simulink model "xfl_em2"  (R2019b)
settings: Solver=FixedStepAuto  StartTime=0  StopTime=50  FixedStep=1e-3  RelTol=1e-3  EnableMultiTasking=on
undefined symbols (not defined in the file or in its folder): qc
libraries: simulink x1
settings Model: Creator=acsl  LastModifiedBy=shawinmihail
settings DataIOCC: LimitDataPoints=on  ReturnWorkspaceOutputs=off
settings OptimizationCC: LifeSpan=inf
settings DebuggingCC: AllowSymbolicDim=off  SFUnexpectedBacktrackingDiag=warning  SFNoUnconditionalDefaultTransitionDiag=warning  SFExecutionAtInitializationDiag=none  ArithmeticOperatorsInVariantConditions=warning
settings ModelReferenceCC: PropagateSignalLabelsOutOfModel=off
settings SFSimCC: SimUseLocalCustomCode=off  CustomCodeUndefinedFunction=UseInterfaceOnly
settings RTWCC: RTWUseLocalCustomCode=off
settings CodeAppCC: StateflowObjectComments=on
settings GRTTargetCC: TargetLangStandard=C89/C90 (ANSI)
settings ConfigComp: CovMetricSettings=dw  CovHtmlReporting=on  CovSaveCumulativeToWorkspaceVar=on  CovSaveSingleToWorkspaceVar=on  CovExternalEMLEnable=off
settings SimscapeCC: SimscapeNormalizeSystem=off
settings ConfigurationSet: Description=SimMechanics 2G

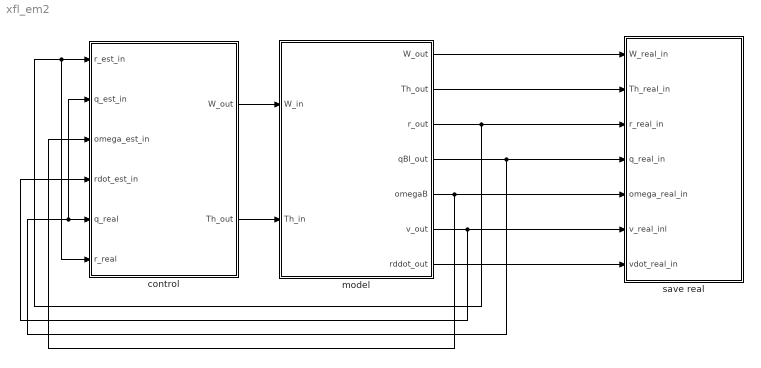
== system xfl_em2 ==
  control : Subsystem  InitFcn=init
  model : Subsystem
  save real : Subsystem
  wires:
  model/2(Th_out) -> save real/2(Th_real_in)
  model/7(rddot_out) -> save real/7(vdot_real_in)
  model/5(omegaB) -> control/3(omega_est_in), save real/5(omega_real_in)
  control/1(W_out) -> model/1(W_in)
  control/2(Th_out) -> model/2(Th_in)
  model/3(r_out) -> control/6(r_real), control/1(r_est_in), save real/3(r_real_in)
  model/4(qBI_out) -> control/5(q_real), control/2(q_est_in), save real/4(q_real_in)
  model/6(v_out) -> control/4(rdot_est_in), save real/6(v_real_inl)
  model/1(W_out) -> save real/1(W_real_in)

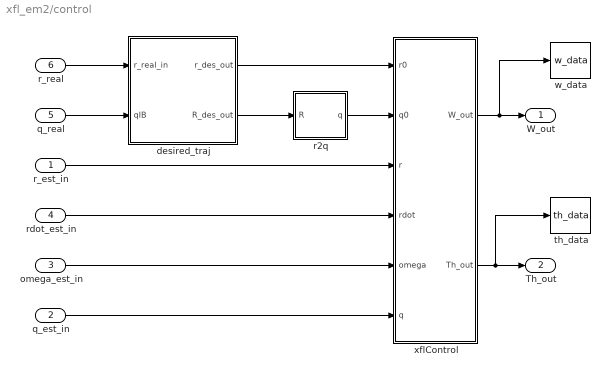
== system xfl_em2/control ==
  r_est_in : Inport
  q_est_in : Inport  Port=2
  omega_est_in : Inport  Port=3
  rdot_est_in : Inport  Port=4
  q_real : Inport  Port=5
  r_real : Inport  Port=6
  desired_traj : Subsystem
  r2q : MATLAB Function  TreatAsAtomicUnit=on
  th_data : ToWorkspace  VariableName=th_data  SaveFormat=Timeseries  SampleTime=-1
  w_data : ToWorkspace  VariableName=w_data  SaveFormat=Timeseries  SampleTime=-1
  xflControl : Subsystem
  W_out : Outport
  Th_out : Outport  Port=2
  wires:
  omega_est_in/1 -> xflControl/5(omega)
  q_est_in/1 -> xflControl/6(q)
  rdot_est_in/1 -> xflControl/4(rdot)
  r_est_in/1 -> xflControl/3(r)
  desired_traj/1(r_des_out) -> xflControl/1(r0)
  desired_traj/2(R_des_out) -> r2q/1(R)
  xflControl/1(W_out) -> w_data/1, W_out/1
  xflControl/2(Th_out) -> th_data/1, Th_out/1
  r2q/1(q) -> xflControl/2(q0)
  r_real/1 -> desired_traj/1(r_real_in)
  q_real/1 -> desired_traj/2(qIB)

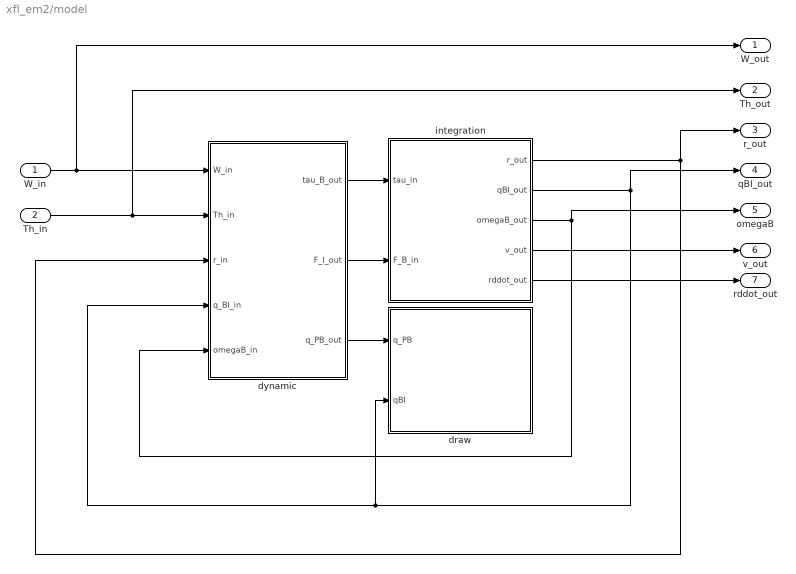
== system xfl_em2/model ==
  W_in : Inport
  Th_in : Inport  Port=2
  draw : Subsystem
  dynamic : Subsystem  StopFcn=close all
  integration : Subsystem
  W_out : Outport
  Th_out : Outport  Port=2
  r_out : Outport  Port=3
  qBI_out : Outport  Port=4
  omegaB : Outport  Port=5
  v_out : Outport  Port=6
  rddot_out : Outport  Port=7
  wires:
  integration/1(r_out) -> dynamic/3(r_in), r_out/1
  dynamic/2(F_I_out) -> integration/2(F_B_in)
  integration/2(qBI_out) -> dynamic/4(q_BI_in), draw/2(qBI), qBI_out/1
  W_in/1 -> W_out/1, dynamic/1(W_in)
  dynamic/1(tau_B_out) -> integration/1(tau_in)
  integration/3(omegaB_out) -> dynamic/5(omegaB_in), omegaB/1
  Th_in/1 -> dynamic/2(Th_in), Th_out/1
  dynamic/3(q_PB_out) -> draw/1(q_PB)
  integration/4(v_out) -> v_out/1
  integration/5(rddot_out) -> rddot_out/1

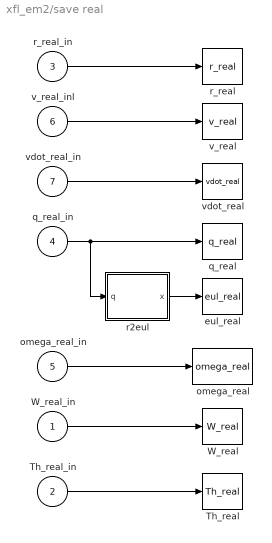
== system xfl_em2/save real ==
  W_real_in : Inport
  Th_real_in : Inport  Port=2
  r_real_in : Inport  Port=3
  q_real_in : Inport  Port=4
  omega_real_in : Inport  Port=5
  v_real_inl : Inport  Port=6
  vdot_real_in : Inport  Port=7
  Th_real : ToWorkspace  VariableName=Th_real  SaveFormat=Timeseries  SampleTime=-1
  W_real : ToWorkspace  VariableName=W_real  SaveFormat=Timeseries  SampleTime=-1
  eul_real : ToWorkspace  VariableName=eul_real  SaveFormat=Timeseries  SampleTime=-1
  omega_real : ToWorkspace  VariableName=omega_real  SaveFormat=Timeseries  SampleTime=-1
  q_real : ToWorkspace  VariableName=q_real  SaveFormat=Timeseries  SampleTime=-1
  r2eul : MATLAB Function  TreatAsAtomicUnit=on
  r_real : ToWorkspace  VariableName=r_real  SaveFormat=Timeseries  SampleTime=-1
  v_real : ToWorkspace  VariableName=v_real  SaveFormat=Timeseries  SampleTime=-1
  vdot_real : ToWorkspace  VariableName=vdot_real  SaveFormat=Timeseries  SampleTime=-1
  wires:
  q_real_in/1 -> q_real/1, r2eul/1(q)
  r_real_in/1 -> r_real/1
  v_real_inl/1 -> v_real/1
  vdot_real_in/1 -> vdot_real/1
  r2eul/1(x) -> eul_real/1
  omega_real_in/1 -> omega_real/1
  Th_real_in/1 -> Th_real/1
  W_real_in/1 -> W_real/1

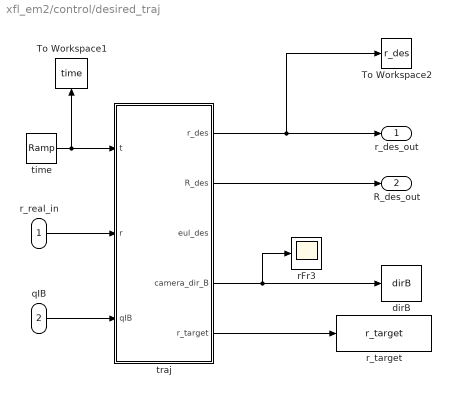
== system xfl_em2/control/desired_traj ==
  r_real_in : Inport
  qIB : Inport  Port=2
  To Workspace1 : ToWorkspace  VariableName=time  SaveFormat=Timeseries  SampleTime=-1
  To Workspace2 : ToWorkspace  VariableName=r_des  SaveFormat=Timeseries  SampleTime=-1
  dirB : ToWorkspace  VariableName=dirB  SaveFormat=Timeseries  SampleTime=-1
  rFr3 : Scope
  r_target : ToWorkspace  VariableName=r_target  SaveFormat=Timeseries  SampleTime=-1
  time : simulink/Sources/Ramp  slope=1  start=0  InitialOutput=0
  traj : MATLAB Function  TreatAsAtomicUnit=on
  r_des_out : Outport
  R_des_out : Outport  Port=2
  wires:
  traj/2(R_des) -> R_des_out/1
  time/1 -> traj/1(t), To Workspace1/1
  r_real_in/1 -> traj/2(r)
  traj/1(r_des) -> To Workspace2/1, r_des_out/1
  qIB/1 -> traj/3(qIB)
  traj/4(camera_dir_B) -> dirB/1, rFr3/1
  traj/5(r_target) -> r_target/1

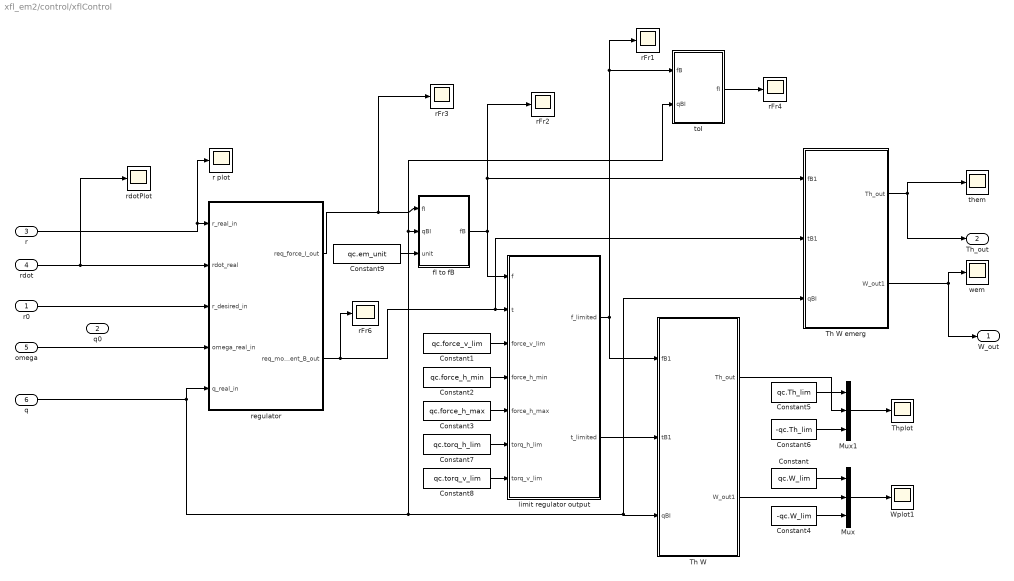
== system xfl_em2/control/xflControl ==
  r0 : Inport
  q0 : Inport  Port=2
  r : Inport  Port=3
  rdot : Inport  Port=4
  omega : Inport  Port=5
  q : Inport  Port=6
  Constant : Constant  Value=qc.W_lim
  Constant1 : Constant  Value=qc.force_v_lim
  Constant2 : Constant  Value=qc.force_h_min
  Constant3 : Constant  Value=qc.force_h_max
  Constant4 : Constant  Value=-qc.W_lim
  Constant5 : Constant  Value=qc.Th_lim
  Constant6 : Constant  Value=-qc.Th_lim
  Constant7 : Constant  Value=qc.torq_h_lim
  Constant8 : Constant  Value=qc.torq_v_lim
  Constant9 : Constant  Value=qc.em_unit
  Mux : Mux  Inputs=3
  Mux1 : Mux  Inputs=3
  Th W : Subsystem
  Th W emerg : Subsystem
  Thplot : Scope
  Wplot1 : Scope
  fI to fB : MATLAB Function  TreatAsAtomicUnit=on
  limit regulator output : MATLAB Function  TreatAsAtomicUnit=on
  r plot : Scope
  rFr{1..4,6} (5 alike) : Scope
  rdotPlot : Scope
  regulator : Subsystem
  them : Scope
  toI : MATLAB Function  TreatAsAtomicUnit=on
  wem : Scope
  W_out : Outport
  Th_out : Outport  Port=2
  wires:
  rdot/1 -> regulator/2(rdot_real), rdotPlot/1
  r0/1 -> regulator/3(r_desired_in)
  r/1 -> r plot/1, regulator/1(r_real_in)
  omega/1 -> regulator/4(omega_real_in)
  Th W/1(Th_out) -> Mux1/2
  Th W/2(W_out1) -> Mux/2
  regulator/1(req_force_I_out) -> rFr3/1, fI to fB/1(fI)
  regulator/2(req_moment_B_out) -> Th W emerg/2(tB1), limit regulator output/2(t), rFr6/1
  q/1 -> regulator/5(q_real_in), Th W emerg/3("qBI "), Th W/3("qBI "), toI/2(qBI), fI to fB/2(qBI)
  Constant/1 -> Mux/1
  Constant4/1 -> Mux/3
  Mux1/1 -> Thplot/1
  Constant5/1 -> Mux1/1
  Constant6/1 -> Mux1/3
  limit regulator output/2(t_limited) -> Th W/2(tB1)
  limit regulator output/1(f_limited) -> toI/1(fB), rFr1/1, Th W/1(fB1)
  Constant1/1 -> limit regulator output/3(force_v_lim)
  Constant2/1 -> limit regulator output/4(force_h_min)
  Constant3/1 -> limit regulator output/5(force_h_max)
  Constant7/1 -> limit regulator output/6(torq_h_lim)
  Constant8/1 -> limit regulator output/7(torq_v_lim)
  fI to fB/1(fB) -> limit regulator output/1(f), rFr2/1, Th W emerg/1(fB1)
  toI/1(fI) -> rFr4/1
  Mux/1 -> Wplot1/1
  Th W emerg/1(Th_out) -> Th_out/1, them/1
  Th W emerg/2(W_out1) -> W_out/1, wem/1
  Constant9/1 -> fI to fB/3(unit)

== system xfl_em2/model/draw ==
  q_PB : Inport
  qBI : Inport  Port=2
  Constant : Constant  Value=qc.rays
  Constant1 : Constant  Value=qc.l
  Constant2 : Constant  Value=qc.draw_mode
  Rate Transition : RateTransition
  Rate Transition1 : RateTransition
  draw : MATLAB Function  TreatAsAtomicUnit=on  SystemSampleTime=qc.draw_tick
  wires:
  Constant1/1 -> draw/4(l)
  q_PB/1 -> Rate Transition1/1
  Rate Transition1/1 -> draw/2(q_PB)
  Constant/1 -> draw/3(rays)
  Rate Transition/1 -> draw/1(q_BI)
  qBI/1 -> Rate Transition/1
  Constant2/1 -> draw/5(draw_mode)

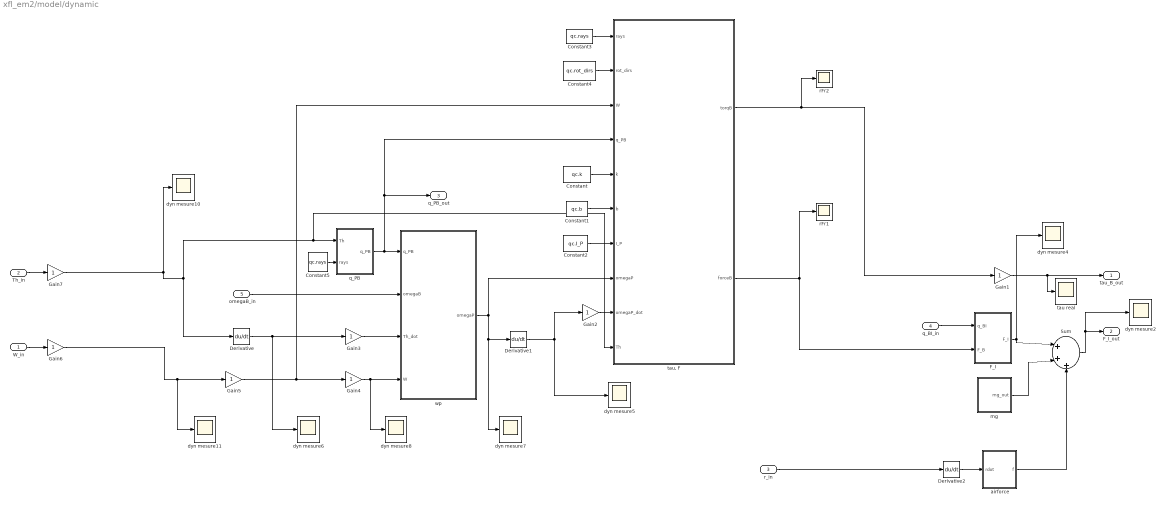
== system xfl_em2/model/dynamic ==
  W_in : Inport
  Th_in : Inport  Port=2
  r_in : Inport  Port=3
  q_BI_in : Inport  Port=4
  omegaB_in : Inport  Port=5
  Constant : Constant  Value=qc.k
  Constant1 : Constant  Value=qc.b
  Constant2 : Constant  Value=qc.I_P
  Constant3 : Constant  Value=qc.rays
  Constant4 : Constant  Value=qc.rot_dirs
  Constant5 : Constant  Value=qc.rays
  Derivative : Derivative
  Derivative1 : Derivative
  Derivative2 : Derivative
  F_I : MATLAB Function  TreatAsAtomicUnit=on
  Gain{1..7} (7 alike) : Gain
  Sum : Sum  Inputs=|+++
  airforce : Subsystem
  dyn mesure{2,4..8,10..11} (8 alike) : Scope
  mg : Subsystem
  q_PB : MATLAB Function  TreatAsAtomicUnit=on
  rFr1 : Scope
  rFr2 : Scope
  tau real : Scope
  "tau, F" : MATLAB Function  TreatAsAtomicUnit=on
  wp : MATLAB Function  TreatAsAtomicUnit=on
  tau_B_out : Outport
  F_I_out : Outport  Port=2
  q_PB_out : Outport  Port=3
  wires:
  q_PB/1(q_PB) -> "tau, F"/4(q_PB), q_PB_out/1, wp/1(q_PB)
  omegaB_in/1 -> wp/2(omegaB)
  Derivative/1 -> dyn mesure6/1, Gain3/1
  wp/1(omegaP) -> dyn mesure7/1, Derivative1/1, "tau, F"/8(omegaP)
  Constant/1 -> "tau, F"/5(k)
  Constant1/1 -> "tau, F"/6(b)
  Constant2/1 -> "tau, F"/7(I_P)
  Constant3/1 -> "tau, F"/1(rays)
  Constant4/1 -> "tau, F"/2(rot_dirs)
  Constant5/1 -> q_PB/2(rays)
  q_BI_in/1 -> F_I/1(q_BI)
  F_I/1(F_I) -> Sum/1, dyn mesure4/1
  mg/1(mg_out) -> Sum/2
  Sum/1 -> dyn mesure2/1, F_I_out/1
  r_in/1 -> Derivative2/1
  airforce/1(f) -> Sum/3
  Derivative2/1 -> airforce/1(rdot)
  Gain2/1 -> "tau, F"/9(omegaP_dot)
  Gain3/1 -> wp/3(Th_dot)
  Gain4/1 -> dyn mesure8/1, wp/4(W)
  Derivative1/1 -> dyn mesure5/1, Gain2/1
  Gain1/1 -> tau_B_out/1, tau real/1
  Gain5/1 -> "tau, F"/3(W), Gain4/1
  Gain6/1 -> dyn mesure11/1, Gain5/1
  Gain7/1 -> "tau, F"/10(Th), q_PB/1(Th), Derivative/1, dyn mesure10/1
  W_in/1 -> Gain6/1
  Th_in/1 -> Gain7/1
  "tau, F"/1(torqB) -> rFr2/1, Gain1/1
  "tau, F"/2(forceB) -> rFr1/1, F_I/2(F_B)

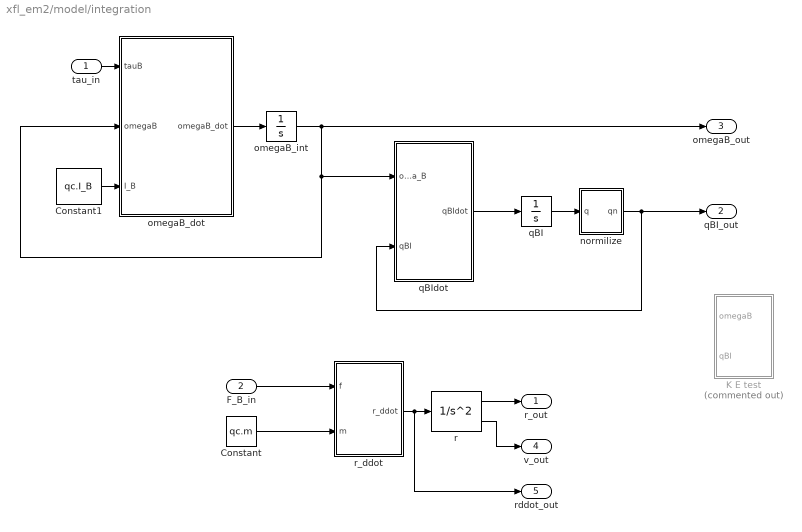
== system xfl_em2/model/integration ==
  tau_in : Inport
  F_B_in : Inport  Port=2
  Constant : Constant  Value=qc.m
  Constant1 : Constant  Value=qc.I_B
  K E test : Subsystem  Commented=on
  normilize : MATLAB Function  TreatAsAtomicUnit=on
  omegaB_dot : MATLAB Function  TreatAsAtomicUnit=on
  omegaB_int : Integrator  InitialCondition=qc.omegaB0
  qBI : Integrator  InitialCondition=qc.qBI0
  qBIdot : MATLAB Function  TreatAsAtomicUnit=on
  r : SecondOrderIntegrator  ICX=qc.r0  ICDXDT=qc.v0
  r_ddot : MATLAB Function  TreatAsAtomicUnit=on
  r_out : Outport
  qBI_out : Outport  Port=2
  omegaB_out : Outport  Port=3
  v_out : Outport  Port=4
  rddot_out : Outport  Port=5
  wires:
  r/1 -> r_out/1
  r_ddot/1(r_ddot) -> rddot_out/1, r/1
  Constant/1 -> r_ddot/2(m)
  omegaB_int/1 -> omegaB_out/1, qBIdot/1(omega_B), omegaB_dot/2(omegaB)
  Constant1/1 -> omegaB_dot/3(I_B)
  tau_in/1 -> omegaB_dot/1(tauB)
  qBIdot/1(qBIdot) -> qBI/1
  qBI/1 -> normilize/1(q)
  normilize/1(qn) -> qBI_out/1, qBIdot/2(qBI)
  F_B_in/1 -> r_ddot/1(f)
  omegaB_dot/1(omegaB_dot) -> omegaB_int/1
  r/2 -> v_out/1

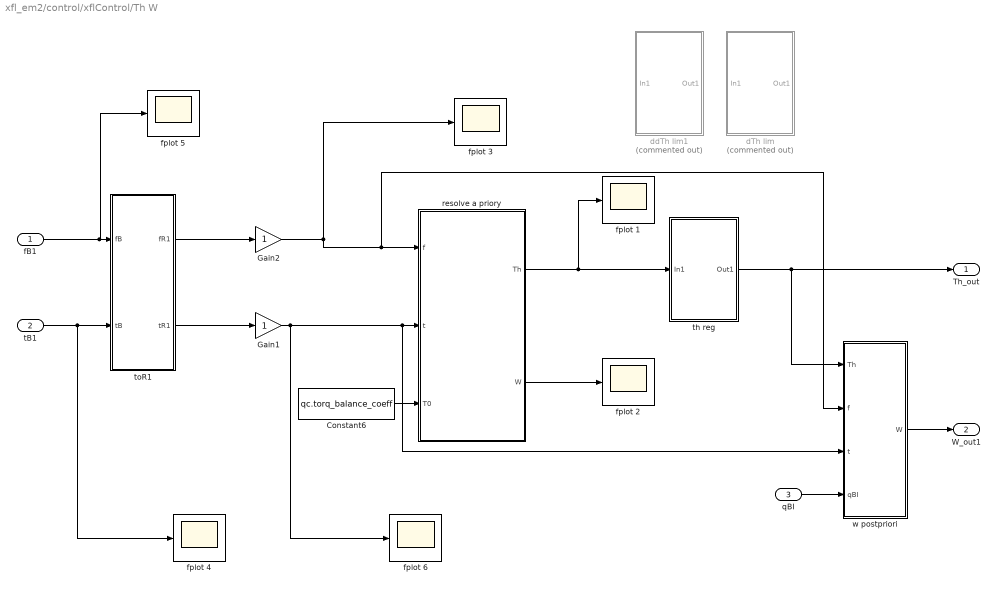
== system xfl_em2/control/xflControl/Th W ==
  fB1 : Inport
  tB1 : Inport  Port=2
  "qBI " : Inport  Port=3
  Constant6 : Constant  Value=qc.torq_balance_coeff
  Gain1 : Gain
  Gain2 : Gain
  dTh lim : Subsystem  Commented=on
  ddTh lim1 : Subsystem  Commented=on
  fplot {1..6} (6 alike) : Scope
  resolve a priory : MATLAB Function  TreatAsAtomicUnit=on
  th reg : Subsystem
  toR1 : MATLAB Function  TreatAsAtomicUnit=on
  w postpriori : MATLAB Function  TreatAsAtomicUnit=on
  Th_out : Outport
  W_out1 : Outport  Port=2
  wires:
  Gain1/1 -> w postpriori/3(t), resolve a priory/2(t), fplot 6/1
  Gain2/1 -> fplot 3/1, w postpriori/2(f), resolve a priory/1(f)
  Constant6/1 -> resolve a priory/3(T0)
  fB1/1 -> fplot 5/1, toR1/1(fB)
  toR1/2(tR1) -> Gain1/1
  toR1/1(fR1) -> Gain2/1
  w postpriori/1(W) -> W_out1/1
  th reg/1(Out1) -> Th_out/1, w postpriori/1(Th)
  resolve a priory/1(Th) -> fplot 1/1, th reg/1(In1)
  "qBI "/1 -> w postpriori/4(qBI)
  resolve a priory/2(W) -> fplot 2/1
  tB1/1 -> fplot 4/1, toR1/2(tB)

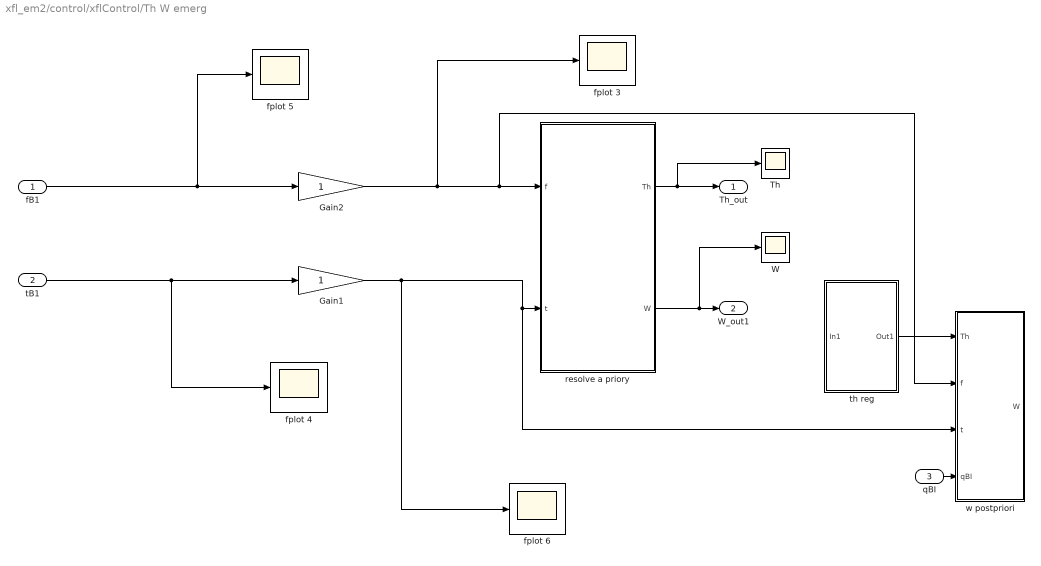
== system xfl_em2/control/xflControl/Th W emerg ==
  fB1 : Inport
  tB1 : Inport  Port=2
  "qBI " : Inport  Port=3
  Gain1 : Gain
  Gain2 : Gain
  Th : Scope
  W : Scope
  fplot {3..6} (4 alike) : Scope
  resolve a priory : MATLAB Function  TreatAsAtomicUnit=on
  th reg : Subsystem
  w postpriori : MATLAB Function  TreatAsAtomicUnit=on
  Th_out : Outport
  W_out1 : Outport  Port=2
  wires:
  Gain1/1 -> w postpriori/3(t), resolve a priory/2(t), fplot 6/1
  Gain2/1 -> fplot 3/1, w postpriori/2(f), resolve a priory/1(f)
  th reg/1(Out1) -> w postpriori/1(Th)
  "qBI "/1 -> w postpriori/4(qBI)
  resolve a priory/2(W) -> W/1, W_out1/1
  resolve a priory/1(Th) -> Th/1, Th_out/1
  tB1/1 -> Gain1/1, fplot 4/1
  fB1/1 -> Gain2/1, fplot 5/1

== system xfl_em2/control/xflControl/regulator ==
  r_real_in : Inport
  rdot_real : Inport  Port=2
  r_desired_in : Inport  Port=3
  omega_real_in : Inport  Port=4
  q_real_in : Inport  Port=5
  Scope3 : Scope
  req torq : Subsystem
  req_force_I : Subsystem
  rgb1 : Scope
  req_force_I_out : Outport
  req_moment_B_out : Outport  Port=2
  wires:
  req_force_I/1(force I out) -> req torq/1(f reg I), req_force_I_out/1, rgb1/1
  r_real_in/1 -> req_force_I/1(r_real_in)
  rdot_real/1 -> req_force_I/2(rdot_real)
  r_desired_in/1 -> req_force_I/3(r_desired_in)
  req torq/1(tB) -> req_moment_B_out/1, Scope3/1
  q_real_in/1 -> req torq/2(q_real_in)
  omega_real_in/1 -> req torq/3(omega_real_in)

== system xfl_em2/model/dynamic/airforce ==
  rdot : Inport
  Constant10 : Constant  Value=qc.S
  Constant8 : Constant  Value=qc.ro
  Constant9 : Constant  Value=qc.c
  air force I : MATLAB Function  TreatAsAtomicUnit=on
  f : Outport
  wires:
  air force I/1(f) -> f/1
  Constant9/1 -> air force I/3(c)
  Constant10/1 -> air force I/4(S)
  Constant8/1 -> air force I/2(ro)
  rdot/1 -> air force I/1(r_dot)

== system xfl_em2/model/dynamic/mg ==
  Constant6 : Constant  Value=qc.m
  Constant7 : Constant  Value=qc.g
  mg : MATLAB Function  TreatAsAtomicUnit=on
  mg_out : Outport
  wires:
  Constant7/1 -> mg/2(g)
  Constant6/1 -> mg/1(m)
  mg/1(mg) -> mg_out/1

== system xfl_em2/model/integration/K E test ==
  omegaB : Inport
  qBI : Inport  Port=2
  Constant2 : Constant  Value=qc.I_B
  "K, E" : MATLAB Function  TreatAsAtomicUnit=on
  rgb : Scope
  rgb1 : Scope
  wires:
  omegaB/1 -> "K, E"/2(omega_B)
  qBI/1 -> "K, E"/3(qBI)
  "K, E"/1(K) -> rgb/1
  "K, E"/2(E) -> rgb1/1
  Constant2/1 -> "K, E"/1(I_B)

== system xfl_em2/control/xflControl/Th W/dTh lim ==
  In1 : Inport
  Constant1 : Constant  Value=1e-2
  Memory : Memory  InitialCondition=[0 0 0 0]'
  fplot 1 : Scope
  thdot limit : MATLAB Function  TreatAsAtomicUnit=on
  Out1 : Outport
  wires:
  thdot limit/2(Th_dot) -> fplot 1/1
  Memory/1 -> thdot limit/2(Th0)
  thdot limit/1(Th_limited) -> Out1/1
  Constant1/1 -> thdot limit/3(dt)
  In1/1 -> thdot limit/1(Th), Memory/1

== system xfl_em2/control/xflControl/Th W/ddTh lim1 ==
  In1 : Inport
  Constant1 : Constant  Value=1e-2
  Memory : Memory  InitialCondition=[0 0 0 0]'
  Memory1 : Memory  InitialCondition=[0 0 0 0]'
  fplot {1..4} (4 alike) : Scope
  thdot limit : MATLAB Function  TreatAsAtomicUnit=on
  Out1 : Outport
  wires:
  thdot limit/3(ddTh) -> fplot 2/1
  Memory1/1 -> thdot limit/2(Th1), Memory/1
  thdot limit/2(dTh1_limited) -> fplot 1/1
  Memory/1 -> thdot limit/3(Th0)
  thdot limit/1(Th_limited) -> Out1/1, fplot 3/1, Memory1/1
  Constant1/1 -> thdot limit/4(dt)
  In1/1 -> thdot limit/1(Th2), fplot 4/1

== system xfl_em2/control/xflControl/Th W/th reg ==
  In1 : Inport
  Memory1 : Memory  InitialCondition=[0 0 0 0]'
  fplot 3 : Scope
  fplot 4 : Scope
  thdot limit : MATLAB Function  TreatAsAtomicUnit=on
  Out1 : Outport
  wires:
  In1/1 -> thdot limit/1(Th_des), fplot 4/1
  Memory1/1 -> thdot limit/2(Th0)
  thdot limit/1(Th) -> Memory1/1, Out1/1, fplot 3/1

== system xfl_em2/control/xflControl/Th W emerg/th reg ==
  In1 : Inport
  Memory1 : Memory  InitialCondition=[0 0 0 0]'
  fplot 3 : Scope
  fplot 4 : Scope
  thdot limit : MATLAB Function  TreatAsAtomicUnit=on
  Out1 : Outport
  wires:
  In1/1 -> thdot limit/1(Th_des), fplot 4/1
  Memory1/1 -> thdot limit/2(Th0)
  thdot limit/1(Th) -> Memory1/1, Out1/1, fplot 3/1

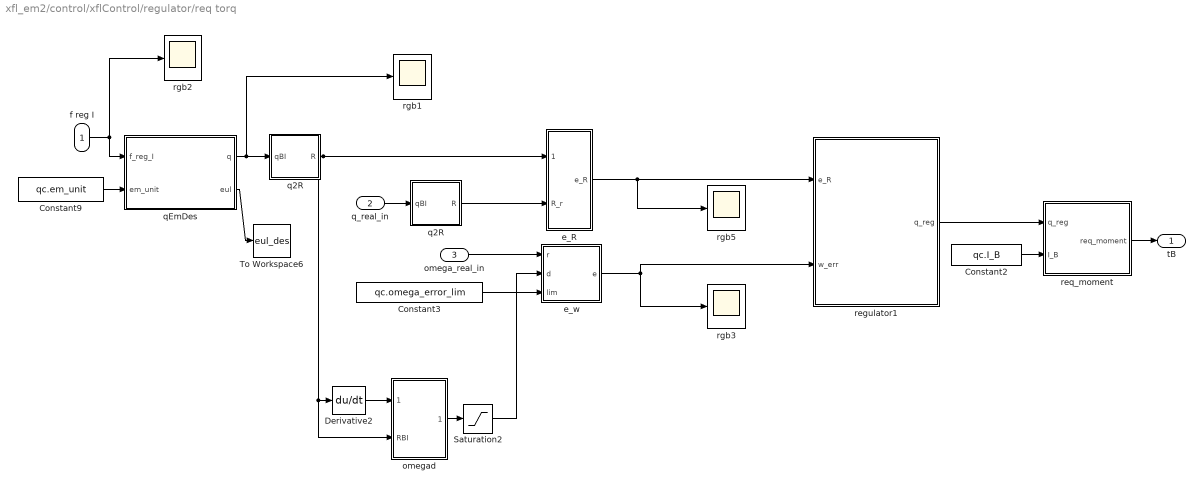
== system xfl_em2/control/xflControl/regulator/req torq ==
  f reg I : Inport
  q_real_in : Inport  Port=2
  omega_real_in : Inport  Port=3
  Constant2 : Constant  Value=qc.I_B
  Constant3 : Constant  Value=qc.omega_error_lim
  Constant9 : Constant  Value=qc.em_unit
  Derivative2 : Derivative
  Saturation2 : Saturate  UpperLimit=qc.w_des_lim  LowerLimit=-qc.w_des_lim
  To Workspace6 : ToWorkspace  VariableName=eul_des  SaveFormat=Timeseries  SampleTime=-1
  e_R : MATLAB Function  TreatAsAtomicUnit=on
  e_w : MATLAB Function  TreatAsAtomicUnit=on
  omegad : MATLAB Function  TreatAsAtomicUnit=on
  q2R : MATLAB Function  TreatAsAtomicUnit=on
  "q2R " : MATLAB Function  TreatAsAtomicUnit=on
  qEmDes : MATLAB Function  TreatAsAtomicUnit=on
  regulator1 : MATLAB Function  TreatAsAtomicUnit=on
  req_moment : MATLAB Function  TreatAsAtomicUnit=on
  rgb{1..3,5} (4 alike) : Scope
  tB : Outport
  wires:
  omega_real_in/1 -> e_w/1(r)
  Saturation2/1 -> e_w/2(d)
  q_real_in/1 -> q2R/1(qBI)
  Constant3/1 -> e_w/3(lim)
  Derivative2/1 -> omegad/1(RBIdot)
  Constant2/1 -> req_moment/2(I_B)
  e_w/1(e) -> regulator1/2(w_err), rgb3/1
  regulator1/1(q_reg) -> req_moment/1(q_reg)
  e_R/1(e_R) -> regulator1/1(e_R), rgb5/1
  omegad/1(omega) -> Saturation2/1
  req_moment/1(req_moment) -> tB/1
  f reg I/1 -> rgb2/1, qEmDes/1(f_reg_I)
  q2R/1(R) -> e_R/2(R_r)
  qEmDes/1(q) -> rgb1/1, "q2R "/1(qBI)
  Constant9/1 -> qEmDes/2(em_unit)
  "q2R "/1(R) -> Derivative2/1, omegad/2(RBI), e_R/1(R_d)
  qEmDes/2(eul) -> To Workspace6/1

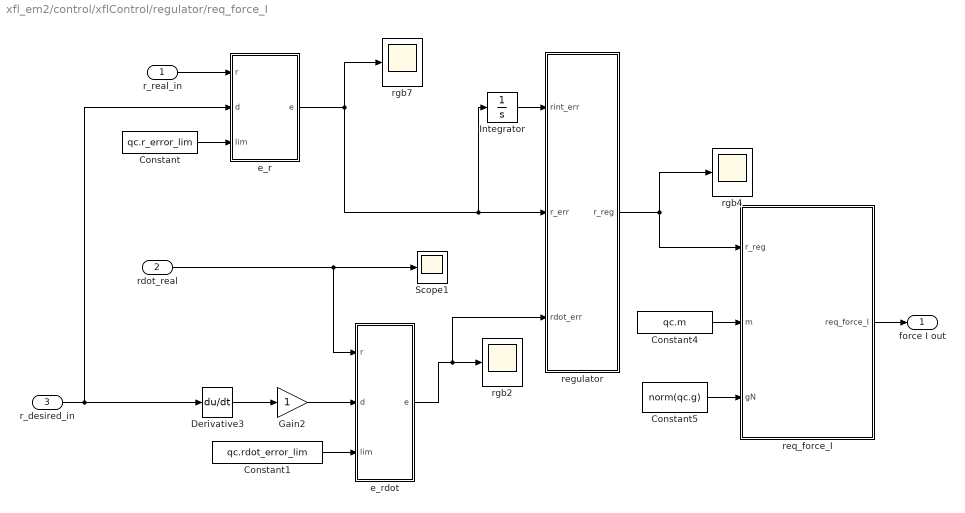
== system xfl_em2/control/xflControl/regulator/req_force_I ==
  r_real_in : Inport
  rdot_real : Inport  Port=2
  r_desired_in : Inport  Port=3
  Constant : Constant  Value=qc.r_error_lim
  Constant1 : Constant  Value=qc.rdot_error_lim
  Constant4 : Constant  Value=qc.m
  Constant5 : Constant  Value=norm(qc.g)
  Derivative3 : Derivative
  Gain2 : Gain
  Integrator : Integrator
  Scope1 : Scope
  e_r : MATLAB Function  TreatAsAtomicUnit=on
  e_rdot : MATLAB Function  TreatAsAtomicUnit=on
  regulator : MATLAB Function  TreatAsAtomicUnit=on
  req_force_I : MATLAB Function  TreatAsAtomicUnit=on
  rgb2 : Scope
  rgb4 : Scope
  rgb7 : Scope
  force I out : Outport
  wires:
  Derivative3/1 -> Gain2/1
  r_real_in/1 -> e_r/1(r)
  r_desired_in/1 -> e_r/2(d), Derivative3/1
  Constant4/1 -> req_force_I/2(m)
  rdot_real/1 -> Scope1/1, e_rdot/1(r)
  e_rdot/1(e) -> rgb2/1, regulator/3(rdot_err)
  regulator/1(r_reg) -> rgb4/1, req_force_I/1(r_reg)
  Constant/1 -> e_r/3(lim)
  Constant1/1 -> e_rdot/3(lim)
  e_r/1(e) -> Integrator/1, regulator/2(r_err), rgb7/1
  Gain2/1 -> e_rdot/2(d)
  req_force_I/1(req_force_I) -> force I out/1
  Integrator/1 -> regulator/1(rint_err)
  Constant5/1 -> req_force_I/3(gN)

== matlab function xfl_em2/model/dynamic/wp ==
  data: q_PB input; omegaP output; omegaB input; Th_dot input; W input
function omegaP  = fcn(q_PB, omegaB, Th_dot, W)

omegaP = zeros(4*3,1);
for i = 1:4
    q_pb = q_PB(:, i);
    q_bp = quatDual(q_pb);
    w = sign(W(i))*sqrt(abs(W(i)));
    omegaP(3*i-2:3*i, 1) = quatRotate(q_bp, omegaB) + [Th_dot(i); 0; w];
end

== matlab function xfl_em2/model/integration/normilize ==
  data: q input; qn output
function qn  = fcn(q)
qn = q / norm(q);

== matlab function xfl_em2/model/dynamic/tau, F ==
  data: torqB output; forceB output; rays input; rot_dirs input; W input; q_PB input; k input; b input; I_P input; omegaP input; omegaP_dot input; Th input
function [torqB, forceB]= fcn(rays, rot_dirs, W, q_PB, k, b, I_P, omegaP, omegaP_dot, Th)

torqB = [0;0;0];
forceB = [0;0;0];

for i = 1:4
    ray = rays(3*i-2:3*i);
    dir = rot_dirs(i);  
    omega_p = omegaP(3*i-2:3*i);
    omega_pz = omega_p(3);
    omega_p_dot = omegaP_dot(3*i-2:3*i);
    q_pb = q_PB(:, i);

    fp = dir * [0;0;k*W(i)];
    fb = quatRotate(q_pb, fp);
        
    tau_p_ext = [0;0;-b*abs(omega_pz)*omega_pz];
    n = 0; %%%%%%% 1 !!!!!!!!!!!!
    tau_p = n*I_P*omega_p_dot + n*cross(omega_p, I_P*omega_p) - tau_p_ext;
    tau_b = cross(ray, fb) - quatRotate(q_pb, tau_p);
    
    torqB = torqB + tau_b;  
    forceB = forceB + fb;
end


% simple dynamic modeling
% J = xfl_J_B(Th(1),Th(2),Th(3),Th(4));
% xdyn = J*W;
% f = xdyn(1:3);
% t = xdyn(4:6);
% 
% torqB = t;
% forceB = f;

== matlab function xfl_em2/control/xflControl/regulator/req torq/e_R ==
  data: R_d input; R_r input; e_R output size=3
function e_R = e_r(R_d, R_r)
Me_R = R_r'*R_d - R_d'*R_r;
e_R = 0.5*[-Me_R(2,3); Me_R(1,3); -Me_R(1,2)];
end

== matlab function xfl_em2/model/dynamic/mg/mg ==
  data: m input; mg output; g input
function mg  = fcn(m, g)
mg = m*g;

== matlab function xfl_em2/model/integration/r_ddot ==
  data: r_ddot output; f input; m input
function r_ddot  = fcn(f, m)

r_ddot = f/m;

== matlab function xfl_em2/save real/r2eul ==
  data: q input; x output
function x = fnc(q)
eul = quat2eul(q');
x = eul';
x = [q(2);q(3);q(4)];
end

== matlab function xfl_em2/model/integration/omegaB_dot ==
  data: tauB input; omegaB_dot output; omegaB input; I_B input
function omegaB_dot  = fcn(tauB, omegaB, I_B)
omegaB_dot = I_B^(-1) * (tauB - 1*cross(omegaB, I_B * omegaB));

== matlab function xfl_em2/model/dynamic/F_I ==
  data: q_BI input; F_I output; F_B input
function F_I  = fcn(q_BI, F_B)
F_I = quatRotate(q_BI, F_B);

== matlab function xfl_em2/model/integration/qBIdot ==
  data: omega_B input; qBIdot output; qBI input
function qBIdot  = fcn(omega_B, qBI)
qw = [0;omega_B];
qBIdot = 0.5*quatMultiply(qBI, qw);

== matlab function xfl_em2/control/xflControl/regulator/req_force_I/e_r ==
  data: r input; d input; e output size=3; lim input
function e = e_r(r, d, lim)
e = d - r;
n = norm(e);
if n < lim
    return;
end
e = lim*e/n;
end

== matlab function xfl_em2/model/draw/draw ==
  data: q_BI input; q_PB input; rays input; l input; draw_mode input
function drawFly(q_BI, q_PB, rays, l, draw_mode)
drawFly(q_BI, q_PB, rays, l, draw_mode)
end

== matlab function xfl_em2/model/integration/K E test/K, E ==
  data: I_B input; omega_B input; qBI input; K output; E output
function [K, E] = fcn(I_B, omega_B, qBI)
K_B = I_B*omega_B;
K = quatRotate(qBI, K_B);
E = omega_B'*I_B*omega_B / 2;

== matlab function xfl_em2/control/xflControl/regulator/req_force_I/e_rdot ==
  data: r input; d input; e output size=3; lim input
function e = e_r(r, d, lim)
e = d - r;
n = norm(e);
if n < lim
    return;
end
e = lim*e/n;
end

== matlab function xfl_em2/control/xflControl/regulator/req torq/e_w ==
  data: r input; d input; e output size=3; lim input
function e = e_r(r, d, lim)
e = d - r;
n = norm(e);
if n < lim
    return;
end
e = lim*e/n;
end

== matlab function xfl_em2/control/xflControl/regulator/req_force_I/regulator ==
  data: rint_err input; r_err input; rdot_err input; r_reg output
function r_reg = x_e(rint_err, r_err, rdot_err)
 
Dr = [1,0,0;
      0,1,0;
      0,0,1]*1;

Pr =   [1,0,0;
       0,1,0;
       0,0,1]*1;
   
Ir =  [1,0,0;
       0,1,0;
       0,0,3]*0;
   
int_lim = 3;
rint_err = min(max(rint_err, -int_lim), int_lim);
 
r_reg =  Dr*(rdot_err)+ Pr*(r_err) + Ir*rint_err;
end

== matlab function xfl_em2/control/xflControl/regulator/req torq/omegad ==
  data: omega output; RBIdot input; RBI input
function omega  = fcn(RBIdot, RBI)

R = RBI'*RBIdot;
omega = [-R(2,3); R(1,3); -R(1,2)];

== matlab function xfl_em2/control/xflControl/regulator/req torq/q2R ==
  data: qBI input; R output
function R = q2R(qBI)
R = quat2matrix(qBI);
end

== matlab function xfl_em2/control/xflControl/limit regulator output ==
  data: f_limited output; f input; t_limited output; t input; force_v_lim input; force_h_min input; force_h_max input; torq_h_lim input; torq_v_lim input
function [f_limited,t_limited]= fcn(f, t, force_v_lim, force_h_min, force_h_max, torq_h_lim, torq_v_lim)

q = [cos(pi/4/2) 0 0 -sin(pi/4/2)]';
f = quatRotate(q, f);
t = quatRotate(q, t);

f_limited = zeros(3,1);
t_limited = zeros(3,1);

f_limited(1) = set_between(f(1), force_v_lim, -force_v_lim);
f_limited(2) = set_between(f(2), force_v_lim, -force_v_lim);
f_limited(3) = set_between(f(3), force_h_max, force_h_min);

t_limited(1) = set_between(t(1), torq_h_lim, -torq_h_lim);
t_limited(2) = set_between(t(2), torq_h_lim, -torq_h_lim);
t_limited(3) = set_between(t(3), torq_v_lim, -torq_v_lim);


q = [cos(pi/4/2) 0 0 sin(pi/4/2)]';
f_limited = quatRotate(q, f_limited);
t_limited = quatRotate(q, t_limited);

end

== matlab function xfl_em2/control/xflControl/regulator/req torq/q2R  ==
  data: qBI input; R output
function R = q2R(qBI)
R = quat2matrix(qBI);
end

== matlab function xfl_em2/control/xflControl/fI to fB ==
  data: fI input; qBI input; fB output; unit input
function fB = q2R(fI, qBI, unit)

fin = fI/norm(fI);
thrB = quatRotate(qBI, unit);
k = dot(thrB, fin);
k = max(0.1, k);
% if k < 0.99
%     k = 0.1;
% end

qIB = quatDual(qBI);
fB = k*quatRotate(qIB, fI);

end

== matlab function xfl_em2/control/xflControl/Th W/toR1 ==
  data: fB input; fR1 output; tB input; tR1 output
function [fR1, tR1]= fcn(fB, tB)
q = [cos(pi/4/2) 0 0 -sin(pi/4/2)]';
fR1 = quatRotate(q, fB);
tR1 = quatRotate(q, tB);
end

== matlab function xfl_em2/control/r2q ==
  data: R input; q output
function q = q2R(R)
q = matrix2quat(R);
end

== matlab function xfl_em2/control/xflControl/regulator/req torq/qEmDes ==
  data: f_reg_I input; q output; em_unit input; eul output
function [q, eul]= fcn(f_reg_I, em_unit)
q = quatBetweenVectors(em_unit, f_reg_I);
eul = [q(2);q(3);q(4)];
end

== matlab function xfl_em2/control/desired_traj/traj ==
  data: r_des output; R_des output; t input; eul_des output; r input; qIB input; camera_dir_B output; r_target output
function [r_des, R_des, eul_des, camera_dir_B, r_target] = curve(t, r, qIB)
r_des = [0;0;0];
s = sqrt(2)/2;
q = [1; 1; -1.3; 2];
q = q / norm(q);
R_des = quat2rotm(q');
eul_des = quat2eul(q')';
camera_dir_B = [0 0 0]';
r_target = [0 0 0]';

end

== matlab function xfl_em2/model/dynamic/q_PB ==
  data: Th input; q_PB output; rays input
function q_PB = fcn(Th, rays)
q_PB = quatPB(Th, rays);
end

== matlab function xfl_em2/model/dynamic/airforce/air force I ==
  data: r_dot input; f output; ro input; c input; S input
function f = fcn(r_dot, ro, c, S)
f = -ro*c*S*norm(r_dot)*r_dot/2;

== matlab function xfl_em2/control/xflControl/Th W/w postpriori ==
  data: Th input; W output; f input; t input; qBI input
function W = fcn(Th, f, t, qBI)

f = quatRotate(quatDual(qBI), f);
R = quat2rotm(qBI');

J = xfl_J_B(Th(1),Th(2),Th(3),Th(4));
J_t = J(4:6, :);
J_f = J(1:3, :);
J_f_I = R * J_f;
A = [J_t; J_f_I(3, :)];

Apinv = pinv(A);
y = [t; f(3)];
W = Apinv*y;

end

== matlab function xfl_em2/control/xflControl/Th W/th reg/thdot limit ==
  data: Th_des input; Th0 input; Th output
function Th = fcn(Th_des, Th0)

dt = 1e-2;
K = 12;
dTh1 = (Th_des - Th0);
Th = Th0 + K*dTh1*dt;


end

== matlab function xfl_em2/control/xflControl/Th W/dTh lim/thdot limit ==
  data: Th input; Th0 input; Th_limited output; Th_dot output; dt input
function [Th_limited, Th_dot]= fcn(Th, Th0, dt)
lim = 5;
dTh = Th - Th0;
Th_dot = dTh ./ dt;
Th_dot = min(max(Th_dot, - lim), lim);
Th_limited = Th0 + Th_dot * dt;
end

== matlab function xfl_em2/control/xflControl/regulator/req torq/regulator1 ==
  data: e_R input; w_err input; q_reg output
function q_reg = x_e(e_R, w_err)
Dq =   [1,0,0;
        0,1,0;
        0,0,1]*12;

Pq =   [1,0,0; 
        0,1,0;
        0,0,1]*12;
          
q_reg = Dq*(w_err) + Pq*(e_R);
end

== matlab function xfl_em2/control/xflControl/Th W/ddTh lim1/thdot limit ==
  data: Th2 input; Th1 input; Th0 input; Th_limited output; dTh1_limited output; dt input; ddTh output
function [Th_limited, dTh1_limited, ddTh]= fcn(Th2, Th1, Th0, dt)

lim = 1;

dTh1 = (Th2 - Th1) / dt;
dTh0 = (Th1 - Th0) / dt;
ddTh = (dTh1 - dTh0) / dt;

ddTh = min(max(ddTh, - lim), lim);
dTh1_limited = dTh0 + ddTh*dt;

Th_limited = Th1 + dTh1_limited * dt + 0.5 * ddTh * dt * dt;
end

== matlab function xfl_em2/control/xflControl/Th W/resolve a priory ==
  data: Th output; f input; W output; t input; T0 input
function [Th, W]= fcn(f, t, T0)
x = [f;t];
%%
tI = 0.5*x(6) + T0;
tII = 0.5*x(6) - T0;

w2 = solutionW2(x(1), x(3)/2, x(4), tII);
th2 = solutionTh2(x(1), x(3)/2, x(4), tII);
w4 = solutionW4(x(1), x(3)/2, x(4), tII);
th4 = solutionTh4(x(1), x(3)/2, x(4), tII);

w1 = solutionW1(x(2), x(3)/2, x(5), tI);
th1 = solutionTh1(x(2), x(3)/2, x(5), tI);
w3 = solutionW3(x(2), x(3)/2, x(5), tI);
th3 = solutionTh3(x(2), x(3)/2, x(5), tI);

W = [w1;w2;w3;w4];
Th = [th1;th2;th3;th4];


% J = xfl_J_B(Th(1),Th(2),Th(3),Th(4));
% xcheck = J*W

end

== matlab function xfl_em2/control/xflControl/regulator/req torq/req_moment ==
  data: q_reg input; req_moment output; I_B input
function req_moment = translate(q_reg, I_B)
req_moment = I_B*q_reg;
end

== matlab function xfl_em2/control/xflControl/Th W emerg/resolve a priory ==
  data: Th output; f input; W output; t input
function [Th, W]= fcn(f, t)

w1 = em_solution_W1(f(1), t(1), t(2), t(3));
th1 = em_solution_Th1(f(1), t(1), t(2), t(3));
w2 = 0;
th2 = 0;
w3 = 0;
th3 = 0;
w4 = em_solution_W4(f(1), t(1), t(2), t(3));
th4 = em_solution_Th4(f(1), t(1), t(2), t(3));

W = [w1;w2;w3;w4];
Th = [th1;th2;th3;th4];

% W = [0;0;0;0];
% Th = [0;0;0;0];

end

== matlab function xfl_em2/control/xflControl/Th W emerg/th reg/thdot limit ==
  data: Th_des input; Th0 input; Th output
function Th = fcn(Th_des, Th0)

dt = 1e-2;
K = 12;
dTh1 = (Th_des - Th0);
Th = Th0 + K*dTh1*dt;


end

== matlab function xfl_em2/control/xflControl/Th W emerg/w postpriori ==
  data: Th input; W output; f input; t input; qBI input
function W = fcn(Th, f, t, qBI)

f = quatRotate(quatDual(qBI), f);
R = quat2rotm(qBI');

J = xfl_J_B(Th(1),Th(2),Th(3),Th(4));
J_t = J(4:6, :);
J_f = J(1:3, :);
J_f_I = R * J_f;
A = [J_t; J_f_I(3, :)];

Apinv = pinv(A);
y = [t; f(3)];
W = Apinv*y;

end

== matlab function xfl_em2/control/xflControl/regulator/req_force_I/req_force_I ==
  data: r_reg input; req_force_I output; m input; gN input
function req_force_I = translate(r_reg, m, gN)
req_force_I = m*r_reg + [0;0;1]*m*gN;
end

== matlab function xfl_em2/control/xflControl/toI ==
  data: fB input; fI output; qBI input
function fI = q2R(fB, qBI)
qIB = quatDual(qBI);
fI = quatRotate(qBI, fB);
end
